simulink model "boost_and_two_level_bridge_sps"  (Simulink 7.6)
settings: Solver=ode23tb  StartTime=0.0  StopTime=0.1  FixedStep=Ts  RelTol=1e-6
PostLoadFcn:
  | Ts = 20e-6;
InitFcn:
  | Ts = 20e-6;
undefined symbols (not defined in the file or in its folder): DiscIntNeverNeededParam, ph
libraries: powerlib x28, rteventslib x6, simulink x1
settings Model: Creator=JeromeCoutel  LastModifiedBy=sebastiencense
settings DebuggingCC: UnconnectedInputMsg=none  UnconnectedOutputMsg=none  UnconnectedLineMsg=none

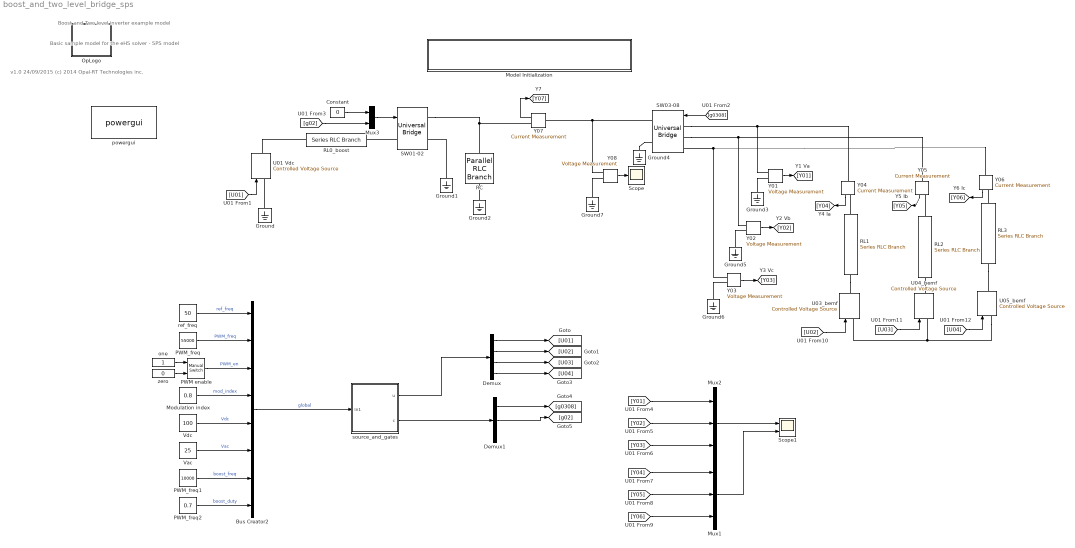
== system boost_and_two_level_bridge_sps ==
  note: v1.0 24/09/2015
      | (c) 2014 Opal-RT Technologies inc.
  note: Boost and Two-level inverter example model
  note: Basic sample model for the eHS solver - SPS model
  Bus Creator2 : BusCreator  Inputs=8
  Constant : Constant  Value=0
  Demux : Demux
  Demux1 : Demux  Outputs=[6 1 -1]
  Ground{,1..7} (8 alike) : powerlib/Elements/Ground  LConnTagsString=a
  Model Initialization : Subsystem  mask(Model Functions){InitFcnX=Ts = 20e-6;, prel=off, posl=on, inif=on, strf=off}
      mask prompts: InitFcnX "Initialisation"; prel "Preload Function"; posl "PostLoad Function"; inif "InitFcn"; strf "StartFcn"
      mask init:
      | currentBlock = gcb;
      | root = bdroot(currentBlock);
      | 
      | if ~strcmp(get_param(root,'BlockDiagramType'),'library')
      |     if prel==1
      |         set_param(root, 'PreLoadFcn', InitFcnX);
      |     else
      |         set_param(root, 'PreLoadFcn', '');
      |     end
      |     if inif==1
      |         set_param(root, 'InitFcn', InitFcnX);
      |     else
      |         set_param(root, 'InitFcn', '');
      |     end
      |     if strf==1
      |         set_param(root, 'StartFcn', InitFcnX);
      |     else
      |         set_param(root, 'StartFcn', '');
      |     end
      |     if posl==1
      |         set_param(root, 'PostLoadFcn', InitFcnX);
      |     else
      |         set_param(root, 'PostLoadFcn', '');
      |     end
      | end
      | 
      | pos = get_param(currentBlock, 'Position');
      | width = pos(3) - pos(1); height = pos(4) - pos(2);
      | txt = [ upper(root) '\n' '- InitFcn. . . . . '  get_param(root, 'InitFcn') ];
      settings: CopyFcn=set_param(gcb,'LinkStatus','none')
      mask Display: text(5, height*0.5, txt, 'horizontalAlignment', 'left', 'verticalAlignment', 'middle') ;
  Modulation index : Constant  Value=0.8
  Mux1 : Mux  Inputs=3
  Mux2 : Mux  Inputs=3
  Mux3 : Mux  Inputs=2
  OpLogo : Subsystem
      mask Display:
      | opLogo = imread('efsOpLogo.tif','tif');
      | image(opLogo(:,:,1:3));
  PWM enable : simulink/Signal Routing/Manual Switch  sw=1  action=0  varsize=off
  PWM_freq : Constant  Value=55000
  PWM_freq1 : Constant  Value=10000
  PWM_freq2 : Constant  Value=0.7
  RC : powerlib/Elements/Parallel RLC Branch  LConnTagsString=a  RConnTagsString=__new0  BranchType=RC  Resistance=1e5  Inductance=1e-3  SetiL0=off  InitialCurrent=0  Capacitance=10e-3  Setx0=off  InitialVoltage=0  Measurements=None
  RL0_boost : powerlib/Elements/Series RLC Branch  LConnTagsString=__new0  RConnTagsString=__new0  BranchType=RL  Resistance=10e-3  Inductance=200e-6  SetiL0=off  InitialCurrent=0  Capacitance=2000e-6  Setx0=off  InitialVoltage=0  Measurements=None
  RL1 : powerlib/Elements/Series RLC Branch  LConnTagsString=__new0  RConnTagsString=__new0  BranchType=RL  Resistance=0.1  Inductance=0.2e-3  SetiL0=off  InitialCurrent=0  Capacitance=2000e-6  Setx0=off  InitialVoltage=0  Measurements=None
  RL2 : powerlib/Elements/Series RLC Branch  LConnTagsString=__new0  RConnTagsString=__new0  BranchType=RL  Resistance=0.1  Inductance=0.2e-3  SetiL0=off  InitialCurrent=0  Capacitance=2000e-6  Setx0=off  InitialVoltage=0  Measurements=None
  RL3 : powerlib/Elements/Series RLC Branch  LConnTagsString=__new0  RConnTagsString=__new0  BranchType=RL  Resistance=0.1  Inductance=0.2e-3  SetiL0=off  InitialCurrent=0  Capacitance=2000e-6  Setx0=off  InitialVoltage=0  Measurements=None
  SW01-02 : powerlib/Power Electronics/Universal Bridge  Arms=1  SnubberResistance=1e5  SnubberCapacitance=inf  Device=IGBT / Diodes  Ron=1e-3  Lon=0  ForwardVoltages="[  0  0  ]"  ForwardVoltage=0  GTOparameters=[ 10e-6 , 20e-6 ]  IGBTparameters=[0, 0]  Measurements=None  Measurements_2=None  converterType=Rectifier
  SW03-08 : powerlib/Power Electronics/Universal Bridge  Arms=3  SnubberResistance=1e5  SnubberCapacitance=inf  Device=IGBT / Diodes  Ron=1e-3  Lon=0  ForwardVoltages="[  0  0  ]"  ForwardVoltage=0  GTOparameters=[ 10e-6 , 20e-6 ]  IGBTparameters=[0, 0]  Measurements=None  Measurements_2=None  converterType=Rectifier
  Scope : Scope
      settings: YMin=290  YMax=400
  Scope1 : Scope  NumInputPorts=2
      settings: YMin=-5~-5  YMax=5~5  SaveName=ScopeData2
  U01 Vdc : powerlib/Electrical Sources/Controlled Voltage Source  Initialize=on  Source_Type=AC  Amplitude=0  Phase=0  Frequency=0  Measurements=None
  U03_bemf : powerlib/Electrical Sources/Controlled Voltage Source  Initialize=on  Source_Type=AC  Amplitude=0  Phase=0  Frequency=0  Measurements=None
  U04_bemf : powerlib/Electrical Sources/Controlled Voltage Source  Initialize=on  Source_Type=AC  Amplitude=0  Phase=0  Frequency=0  Measurements=None
  U05_bemf : powerlib/Electrical Sources/Controlled Voltage Source  Initialize=on  Source_Type=AC  Amplitude=0  Phase=0  Frequency=0  Measurements=None
  Vac : Constant  Value=25
  Vdc : Constant  Value=100
  Y01 : powerlib/Measurements/Voltage Measurement  PhasorSimulation=off  OutputType=Complex  PSBequivalent=0
  Y02 : powerlib/Measurements/Voltage Measurement  PhasorSimulation=off  OutputType=Complex  PSBequivalent=0
  Y03 : powerlib/Measurements/Voltage Measurement  PhasorSimulation=off  OutputType=Complex  PSBequivalent=0
  Y04 : powerlib/Measurements/Current Measurement  PhasorSimulation=off  OutputType=Complex  PSBequivalent=0
  Y05 : powerlib/Measurements/Current Measurement  PhasorSimulation=off  OutputType=Complex  PSBequivalent=0
  Y06 : powerlib/Measurements/Current Measurement  PhasorSimulation=off  OutputType=Complex  PSBequivalent=0
  Y07 : powerlib/Measurements/Current Measurement  PhasorSimulation=off  OutputType=Complex  PSBequivalent=0
  Y08 : powerlib/Measurements/Voltage Measurement  PhasorSimulation=off  OutputType=Complex  PSBequivalent=0
  one : Constant
  powergui : powerlib/powergui  Priority=1  SimulationMode=Continuous  SolverType=Tustin  SampleTime=Ts  frequency=60  SPID=off  DisableSnubberDevices=off  DisableRonSwitches=off  DisableVfSwitches=off  SwTol=0  Interpol=off  DisplayEquations=off  FunctionMessages=off  frequencyindice=0  Pbase=100e6  ErrMax=1e-4  Iterations=50  UnitsV=kV  UnitsW=MW  echomessages=off  HookPort=off  EnableUseOfTLC=off  x0status=blocks  RestoreLinks=warning  ResistiveCurrentMeasurement=off  Frange=[0:2:500]  Ylog=off  Xlog=on  ShowGrid=off  save=off  variable=ZData  structure=ScopeData  ZoomFFT=off  StartTime=7.29  cycles=3  DisplayStyle=1  fundamental=50  FreqAxis=off  MaxFrequency=1000  frequencyindicesteady=1  RmsSteady=1  display=off  Ts=0  methode=off
  ref_freq : Constant  Value=50
  source_and_gates : Subsystem
  zero : Constant  Value=0
  wires:
  Y07/1 -> [Y07]
  [U01] -> U01 Vdc/1
  Y06/1 -> [Y06]
  Y04/1 -> [Y04]
  Y05/1 -> [Y05]
  Y01/1 -> [Y01]
  Y03/1 -> [Y03]
  Y02/1 -> [Y02]
  [U02] -> U03_bemf/1
  [U03] -> U04_bemf/1
  [U04] -> U05_bemf/1
  Bus Creator2/1 -> source_and_gates/1(In1)  "global"
  ref_freq/1 -> Bus Creator2/1  "ref_freq"
  PWM_freq/1 -> Bus Creator2/2  "PWM_freq"
  PWM enable/1 -> Bus Creator2/3  "PWM_en"
  Vdc/1 -> Bus Creator2/5  "Vdc"
  zero/1 -> PWM enable/2
  one/1 -> PWM enable/1
  Modulation index/1 -> Bus Creator2/4  "mod_index"
  Vac/1 -> Bus Creator2/6  "Vac"
  source_and_gates/1(u) -> Demux/1
  Demux/1 -> [U01]
  Demux/2 -> [U02]
  Demux/3 -> [U03]
  Demux/4 -> [U04]
  Demux1/1 -> [g0308]
  source_and_gates/2(c) -> Demux1/1
  Demux1/2 -> [g02]
  [g0308] -> SW03-08/1
  Y08/1 -> Scope/1
  Mux2/1 -> Scope1/1
  Mux1/1 -> Scope1/2
  [Y01] -> Mux2/1
  [Y02] -> Mux2/2
  [Y03] -> Mux2/3
  [Y04] -> Mux1/1
  [Y05] -> Mux1/2
  [Y06] -> Mux1/3
  PWM_freq1/1 -> Bus Creator2/7  "boost_freq"
  PWM_freq2/1 -> Bus Creator2/8  "boost_duty"
  Mux3/1 -> SW01-02/1
  [g02] -> Mux3/2
  Constant/1 -> Mux3/1
  connections:
  Y03/LConn1 -- Y06/LConn1 -- SW03-08/LConn3
  RL2/LConn1 -- Y05/RConn1
  RL1/LConn1 -- Y04/RConn1
  RL3/LConn1 -- Y06/RConn1
  Ground/LConn1 -- U01 Vdc/LConn1
  RL3/RConn1 -- U05_bemf/RConn1
  RL2/RConn1 -- U04_bemf/RConn1
  RL1/RConn1 -- U03_bemf/RConn1
  U05_bemf/LConn1 -- U04_bemf/LConn1 -- U03_bemf/LConn1
  Ground5/LConn1 -- Y02/LConn2
  Ground6/LConn1 -- Y03/LConn2
  Ground1/LConn1 -- SW01-02/RConn2
  Ground2/LConn1 -- RC/LConn1
  SW03-08/RConn2 -- Ground4/LConn1
  Ground7/LConn1 -- Y08/LConn2
  RL0_boost/RConn1 -- U01 Vdc/RConn1
  SW01-02/LConn1 -- RL0_boost/LConn1
  SW03-08/LConn1 -- Y01/LConn1 -- Y04/LConn1
  Ground3/LConn1 -- Y01/LConn2
  SW03-08/LConn2 -- Y02/LConn1 -- Y05/LConn1
  RC/RConn1 -- Y07/RConn1 -- SW01-02/RConn1
  SW03-08/RConn1 -- Y08/LConn1 -- Y07/LConn1

== system boost_and_two_level_bridge_sps/Model Initialization ==

== system boost_and_two_level_bridge_sps/OpLogo ==

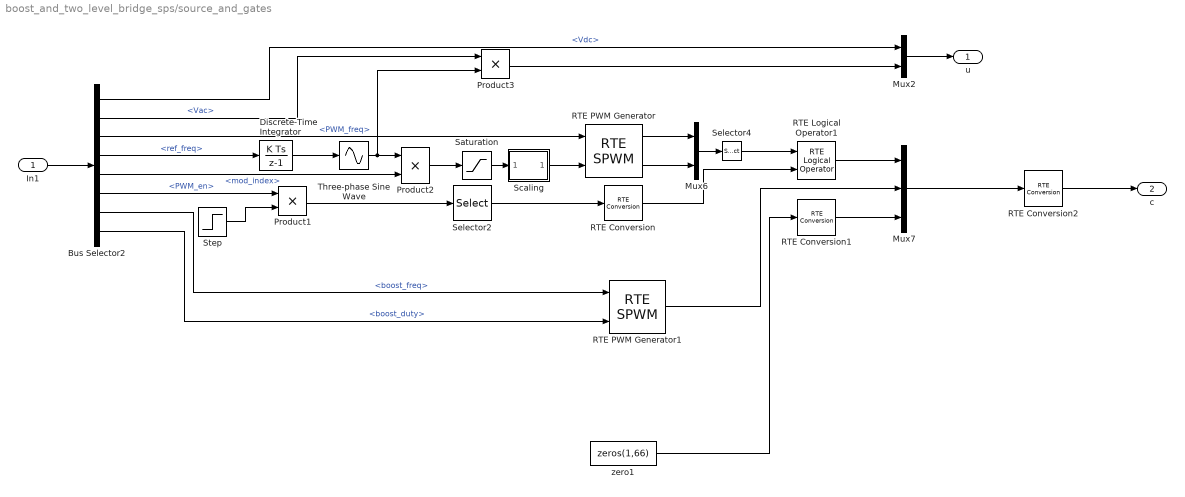
== system boost_and_two_level_bridge_sps/source_and_gates ==
  In1 : Inport
  Bus Selector2 : BusSelector  OutputSignals=Vdc,Vac,PWM_freq,ref_freq,mod_index,PWM_en,boost_freq,boost_duty
  Discrete-Time Integrator : DiscreteIntegrator  gainval=2*pi  SampleTime=20e-6  ICPrevOutput=DiscIntNeverNeededParam  ICPrevScaledInput=DiscIntNeverNeededParam
  Mux2 : Mux  Inputs=2
  Mux6 : Mux  Inputs=2
  Mux7 : Mux  Inputs=[6 1 -1]
  Product1 : Product  RndMeth=Zero
  Product2 : Product  RndMeth=Zero
  Product3 : Product  RndMeth=Zero
  RTE Conversion : rteventslib/Signal Attributes/RTE Conversion  inputdatatype=Double  outputdatatype=RTE Boolean  compensation=Enabled  nbMaxEvents=4  sampleTime=Ts
  RTE Conversion1 : rteventslib/Signal Attributes/RTE Conversion  inputdatatype=Double  outputdatatype=RTE Boolean  compensation=Enabled  nbMaxEvents=4  sampleTime=Ts
  RTE Conversion2 : rteventslib/Signal Attributes/RTE Conversion  inputdatatype=RTE Boolean  outputdatatype=Double  compensation=Disabled  nbMaxEvents=4  sampleTime=Ts
  RTE Logical Operator1 : rteventslib/Math Operations/RTE Logical Operator  LogicalOperator=AND  NbrInput=2  NbrMaxEvents=4
  RTE PWM Generator : rteventslib/Sources/RTE SPWM  NumberPhases=3-ph  CenterAlignmentMode=On  MaxFreq=100e3  MinFreq=0  EnablingPort=off  ComplementaryMode=on  SpaceVector=off  RiseTimeDelay=1e-6  MaxEvents=4  SampleTime=Ts
  RTE PWM Generator1 : rteventslib/Sources/RTE SPWM  NumberPhases=1-ph  CenterAlignmentMode=On  MaxFreq=100e3  MinFreq=0  EnablingPort=off  ComplementaryMode=off  SpaceVector=off  RiseTimeDelay=1e-6  MaxEvents=4  SampleTime=Ts
  Saturation : Saturate  UpperLimit=1  LowerLimit=-1
  Scaling : Subsystem
  Selector2 : Selector  InputPortWidth=1  IndexOptions=Index vector (dialog)  Indices=[ones(1,6)*1]  OutputSizes=1
  Selector4 : Selector  IndexOptions=Index vector (dialog)  Indices=[1 4 2 5 3 6]  OutputSizes=[(-2)]
  Step : Step  Time=0  SampleTime=Ts
  Three-phase Sine Wave : Sin  TimeSource=Use external signal  Phase=[0 -2*pi/3 2*pi/3]
  zero1 : Constant  Value=zeros(1,66)
  u : Outport
  c : Outport  Port=2
  wires:
  RTE Logical Operator1/1 -> Mux7/1
  zero1/1 -> RTE Conversion1/1
  RTE Conversion1/1 -> Mux7/3
  Product3/1 -> Mux2/2
  Bus Selector2/2 -> Product3/1  "<Vac>"
  Mux7/1 -> RTE Conversion2/1
  In1/1 -> Bus Selector2/1
  Mux2/1 -> u/1
  Scaling/1(Out1) -> RTE PWM Generator/2
  Selector4/1 -> RTE Logical Operator1/1
  Bus Selector2/5 -> Product2/2  "<mod_index>"
  Discrete-Time Integrator/1 -> Three-phase Sine Wave/1
  Product1/1 -> Selector2/1
  Product2/1 -> Saturation/1
  Three-phase Sine Wave/1 -> Product3/2, Product2/1
  Saturation/1 -> Scaling/1(In1)
  Mux6/1 -> Selector4/1
  RTE PWM Generator/2 -> Mux6/2
  RTE PWM Generator/1 -> Mux6/1
  RTE Conversion/1 -> RTE Logical Operator1/2
  Selector2/1 -> RTE Conversion/1
  Step/1 -> Product1/2
  Bus Selector2/1 -> Mux2/1  "<Vdc>"
  Bus Selector2/6 -> Product1/1  "<PWM_en>"
  Bus Selector2/4 -> Discrete-Time Integrator/1  "<ref_freq>"
  Bus Selector2/3 -> RTE PWM Generator/1  "<PWM_freq>"
  RTE Conversion2/1 -> c/1
  Bus Selector2/7 -> RTE PWM Generator1/1  "<boost_freq>"
  Bus Selector2/8 -> RTE PWM Generator1/2  "<boost_duty>"
  RTE PWM Generator1/1 -> Mux7/2

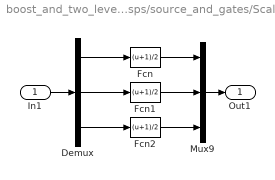
== system boost_and_two_level_bridge_sps/source_and_gates/Scaling ==
  In1 : Inport
  Demux : Demux  Outputs=3
  Fcn : Fcn  Expr=(u+1)/2
  Fcn1 : Fcn  Expr=(u+1)/2
  Fcn2 : Fcn  Expr=(u+1)/2
  Mux9 : Mux  Inputs=3
  Out1 : Outport
  wires:
  Fcn/1 -> Mux9/1
  Fcn1/1 -> Mux9/2
  Fcn2/1 -> Mux9/3
  Mux9/1 -> Out1/1
  Demux/1 -> Fcn/1
  Demux/2 -> Fcn1/1
  Demux/3 -> Fcn2/1
  In1/1 -> Demux/1
